simulink library "host_library"  (R2013b)
settings: Solver=ode45  StartTime=0.0  StopTime=10.0  RelTol=1e-3
libraries: embdlinuxlib x9
settings Model: Creator=scastro  LastModifiedBy=scastro

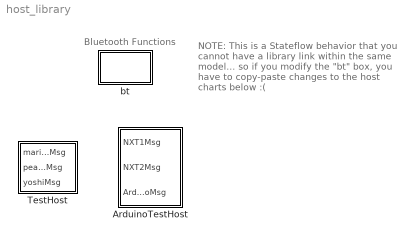
== system host_library ==
  note: NOTE:  This is a Stateflow behavior
      | that you cannot have a library link within the
      | same model... so if you modify the "bt" box,
      | you have to copy-paste changes to the host
      | charts below :(
  note: Bluetooth Functions
  ArduinoTestHost : Stateflow chart  TreatAsAtomicUnit=on
  TestHost : Stateflow chart  TreatAsAtomicUnit=on
  bt : Stateflow chart  TreatAsAtomicUnit=on

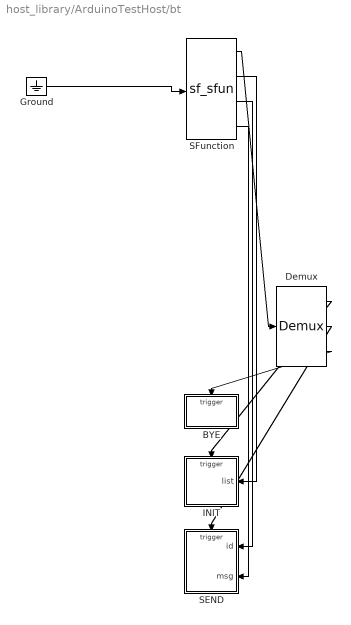
== system host_library/ArduinoTestHost/bt ==
  " Demux " : Demux  Outputs=3
  " Ground " : Ground
  " SFunction " : S-Function  Tag=Stateflow S-Function host_library 4  FunctionName=sf_sfun  PortCounts=[1 4]  EnableBusSupport=off
  BYE : Subsystem
      settings: UndoDeleteFcn=Stateflow.SLINSF.SimulinkMan.restorePreDeleteFcn  PreDeleteFcn=Stateflow.SLINSF.SimulinkMan.removePreDeleteFcn
  INIT : Subsystem
      settings: UndoDeleteFcn=Stateflow.SLINSF.SimulinkMan.restorePreDeleteFcn  PreDeleteFcn=Stateflow.SLINSF.SimulinkMan.removePreDeleteFcn
  SEND : Subsystem
      settings: UndoDeleteFcn=Stateflow.SLINSF.SimulinkMan.restorePreDeleteFcn  PreDeleteFcn=Stateflow.SLINSF.SimulinkMan.removePreDeleteFcn
  wires:
  " SFunction "/1 -> " Demux "/1
  " Ground "/1 -> " SFunction "/1
  " Demux "/3 -> BYE/Trigger
  " Demux "/2 -> SEND/Trigger
  " SFunction "/4 -> SEND/2(msg)
  " SFunction "/3 -> SEND/1(id)
  " Demux "/1 -> INIT/Trigger
  " SFunction "/2 -> INIT/1(list)

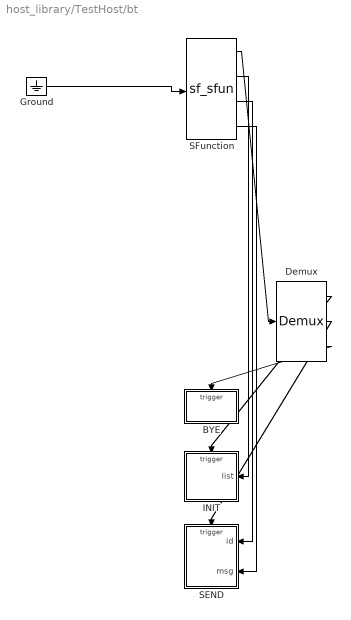
== system host_library/TestHost/bt ==
  " Demux " : Demux  Outputs=3
  " Ground " : Ground
  " SFunction " : S-Function  Tag=Stateflow S-Function host_library 8  FunctionName=sf_sfun  PortCounts=[1 4]  EnableBusSupport=off
  BYE : Subsystem
      settings: UndoDeleteFcn=Stateflow.SLINSF.SimulinkMan.restorePreDeleteFcn  PreDeleteFcn=Stateflow.SLINSF.SimulinkMan.removePreDeleteFcn
  INIT : Subsystem
      settings: UndoDeleteFcn=Stateflow.SLINSF.SimulinkMan.restorePreDeleteFcn  PreDeleteFcn=Stateflow.SLINSF.SimulinkMan.removePreDeleteFcn
  SEND : Subsystem
      settings: UndoDeleteFcn=Stateflow.SLINSF.SimulinkMan.restorePreDeleteFcn  PreDeleteFcn=Stateflow.SLINSF.SimulinkMan.removePreDeleteFcn
  wires:
  " SFunction "/2 -> INIT/1(list)
  " Demux "/1 -> INIT/Trigger
  " SFunction "/3 -> SEND/1(id)
  " SFunction "/4 -> SEND/2(msg)
  " Demux "/2 -> SEND/Trigger
  " Demux "/3 -> BYE/Trigger
  " Ground "/1 -> " SFunction "/1
  " SFunction "/1 -> " Demux "/1

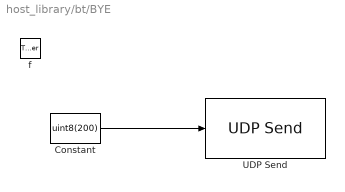
== system host_library/bt/BYE ==
  f : TriggerPort  TriggerType=function-call
      settings: CopyFcn=Stateflow.SLINSF.SimulinkMan.removeBlockPreDeleteFcn  PreDeleteFcn=Stateflow.SLINSF.SimulinkMan.unsafePredeleteFcn
  Constant : Constant  Value=uint8(200)  VectorParams1D=off
      settings: SamplingMode=Frame based
  UDP Send : embdlinuxlib/UDP Send  remoteURL='127.0.0.1'  remotePort=35712  localURL='255.255.255.255'  localPortSource=Automatically determine  localPort=-1  sampletime=-1  blockPlatform=Raspberry Pi  separateLengthPort=0
  wires:
  Constant/1 -> UDP Send/1

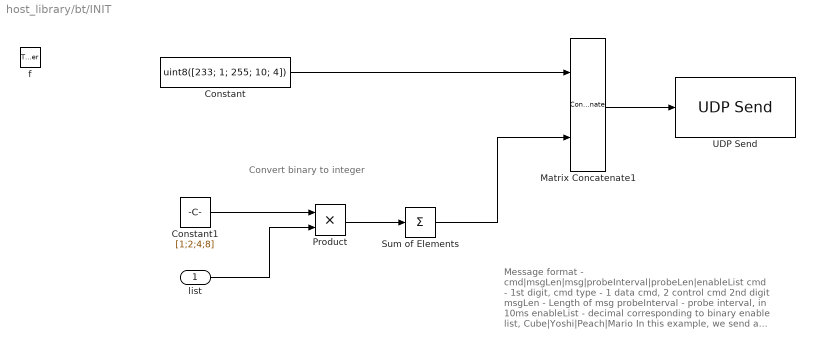
== system host_library/bt/INIT ==
  note: Convert binary to integer
  note: Message format -
      | cmd|msgLen|msg|probeInterval|probeLen|enableList
      | cmd - 1st digit, cmd type - 1 data cmd, 2 control cmd
      | 2nd digit
      | msgLen - Length of msg
      | probeInterval - probe interval, in 10ms
      | enableList - decimal corresponding to binary enable list,
      | Cube|Yoshi|Peach|Mario
      | In this example, we send a unint8 255
  list : Inport  OutDataTypeStr=double  PortDimensions=4
  f : TriggerPort  TriggerType=function-call
      settings: CopyFcn=Stateflow.SLINSF.SimulinkMan.removeBlockPreDeleteFcn  PreDeleteFcn=Stateflow.SLINSF.SimulinkMan.unsafePredeleteFcn
  Constant : Constant  Value=uint8([233; 1; 255; 10; 4])  VectorParams1D=off
      settings: SamplingMode=Frame based
  Constant1 : Constant  Value=[1;2;4;8]
  Matrix Concatenate1 : Concatenate  Mode=Multidimensional array
  Product : Product
  Sum of Elements : Sum  Inputs=+  AccumDataTypeStr=uint8  OutDataTypeStr=uint8
  UDP Send : embdlinuxlib/UDP Send  remoteURL='127.0.0.1'  remotePort=35712  localURL='255.255.255.255'  localPortSource=Automatically determine  localPort=-1  sampletime=-1  blockPlatform=Raspberry Pi  separateLengthPort=0
  wires:
  Matrix Concatenate1/1 -> UDP Send/1
  Constant/1 -> Matrix Concatenate1/1
  Sum of Elements/1 -> Matrix Concatenate1/2
  Product/1 -> Sum of Elements/1
  Constant1/1 -> Product/1
  list/1 -> Product/2

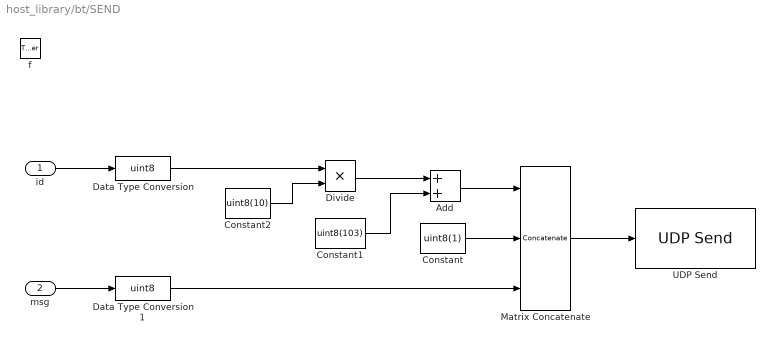
== system host_library/bt/SEND ==
  id : Inport  OutDataTypeStr=Enum: RobotID  PortDimensions=1
  msg : Inport  Port=2  OutDataTypeStr=Enum: StatusID  PortDimensions=1
  f : TriggerPort  TriggerType=function-call
      settings: CopyFcn=Stateflow.SLINSF.SimulinkMan.removeBlockPreDeleteFcn  PreDeleteFcn=Stateflow.SLINSF.SimulinkMan.unsafePredeleteFcn
  Add : Sum
  Constant : Constant  Value=uint8(1)  VectorParams1D=off
  Constant1 : Constant  Value=uint8(103)  VectorParams1D=off
  Constant2 : Constant  Value=uint8(10)  VectorParams1D=off
  Data Type Conversion : DataTypeConversion  OutDataTypeStr=uint8
  Data Type Conversion1 : DataTypeConversion  OutDataTypeStr=uint8
  Divide : Product  Inputs=**  OutDataTypeStr=uint8
  Matrix Concatenate : Concatenate  NumInputs=3  Mode=Multidimensional array
  UDP Send : embdlinuxlib/UDP Send  remoteURL='127.0.0.1'  remotePort=35712  localURL='255.255.255.255'  localPortSource=Automatically determine  localPort=-1  sampletime=-1  blockPlatform=Raspberry Pi  separateLengthPort=0
  wires:
  Matrix Concatenate/1 -> UDP Send/1
  msg/1 -> Data Type Conversion1/1
  Constant/1 -> Matrix Concatenate/2
  Constant2/1 -> Divide/2
  Constant1/1 -> Add/2
  id/1 -> Data Type Conversion/1
  Divide/1 -> Add/1
  Add/1 -> Matrix Concatenate/1
  Data Type Conversion/1 -> Divide/1
  Data Type Conversion1/1 -> Matrix Concatenate/3

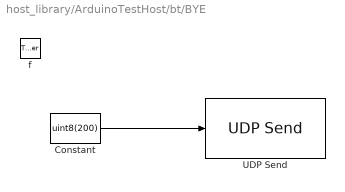
== system host_library/ArduinoTestHost/bt/BYE ==
  f : TriggerPort  TriggerType=function-call
      settings: CopyFcn=Stateflow.SLINSF.SimulinkMan.removeBlockPreDeleteFcn  PreDeleteFcn=Stateflow.SLINSF.SimulinkMan.unsafePredeleteFcn
  Constant : Constant  Value=uint8(200)  VectorParams1D=off
      settings: SamplingMode=Frame based
  UDP Send : embdlinuxlib/UDP Send  remoteURL='127.0.0.1'  remotePort=35712  localURL='255.255.255.255'  localPortSource=Automatically determine  localPort=-1  sampletime=-1  blockPlatform=Raspberry Pi  separateLengthPort=0
  wires:
  Constant/1 -> UDP Send/1

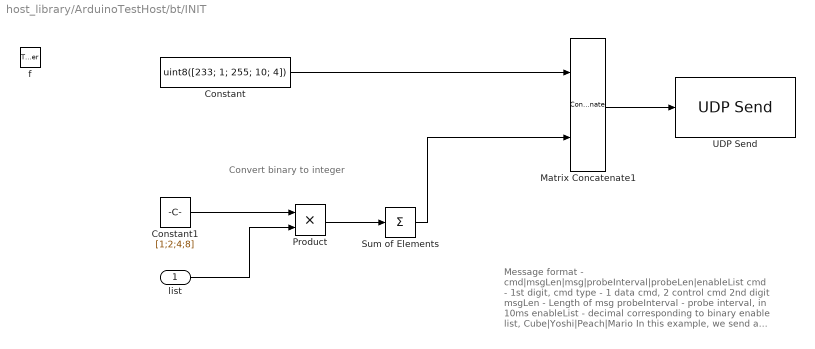
== system host_library/ArduinoTestHost/bt/INIT ==
  note: Convert binary to integer
  note: Message format -
      | cmd|msgLen|msg|probeInterval|probeLen|enableList
      | cmd - 1st digit, cmd type - 1 data cmd, 2 control cmd
      | 2nd digit
      | msgLen - Length of msg
      | probeInterval - probe interval, in 10ms
      | enableList - decimal corresponding to binary enable list,
      | Cube|Yoshi|Peach|Mario
      | In this example, we send a unint8 255
  list : Inport  OutDataTypeStr=double  PortDimensions=4
  f : TriggerPort  TriggerType=function-call
      settings: CopyFcn=Stateflow.SLINSF.SimulinkMan.removeBlockPreDeleteFcn  PreDeleteFcn=Stateflow.SLINSF.SimulinkMan.unsafePredeleteFcn
  Constant : Constant  Value=uint8([233; 1; 255; 10; 4])  VectorParams1D=off
      settings: SamplingMode=Frame based
  Constant1 : Constant  Value=[1;2;4;8]
  Matrix Concatenate1 : Concatenate  Mode=Multidimensional array
  Product : Product
  Sum of Elements : Sum  Inputs=+  AccumDataTypeStr=uint8  OutDataTypeStr=uint8
  UDP Send : embdlinuxlib/UDP Send  remoteURL='127.0.0.1'  remotePort=35712  localURL='255.255.255.255'  localPortSource=Automatically determine  localPort=-1  sampletime=-1  blockPlatform=Raspberry Pi  separateLengthPort=0
  wires:
  list/1 -> Product/2
  Constant1/1 -> Product/1
  Product/1 -> Sum of Elements/1
  Matrix Concatenate1/1 -> UDP Send/1
  Constant/1 -> Matrix Concatenate1/1
  Sum of Elements/1 -> Matrix Concatenate1/2

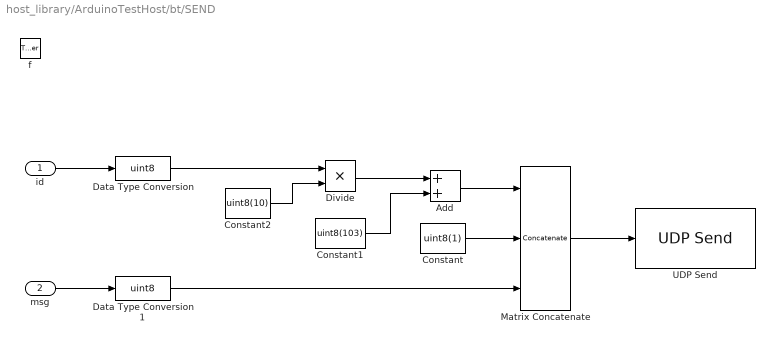
== system host_library/ArduinoTestHost/bt/SEND ==
  id : Inport  OutDataTypeStr=Enum: RobotID  PortDimensions=1
  msg : Inport  Port=2  OutDataTypeStr=Enum: StatusID  PortDimensions=1
  f : TriggerPort  TriggerType=function-call
      settings: CopyFcn=Stateflow.SLINSF.SimulinkMan.removeBlockPreDeleteFcn  PreDeleteFcn=Stateflow.SLINSF.SimulinkMan.unsafePredeleteFcn
  Add : Sum
  Constant : Constant  Value=uint8(1)  VectorParams1D=off
  Constant1 : Constant  Value=uint8(103)  VectorParams1D=off
  Constant2 : Constant  Value=uint8(10)  VectorParams1D=off
  Data Type Conversion : DataTypeConversion  OutDataTypeStr=uint8
  Data Type Conversion1 : DataTypeConversion  OutDataTypeStr=uint8
  Divide : Product  Inputs=**  OutDataTypeStr=uint8
  Matrix Concatenate : Concatenate  NumInputs=3  Mode=Multidimensional array
  UDP Send : embdlinuxlib/UDP Send  remoteURL='127.0.0.1'  remotePort=35712  localURL='255.255.255.255'  localPortSource=Automatically determine  localPort=-1  sampletime=-1  blockPlatform=Raspberry Pi  separateLengthPort=0
  wires:
  Matrix Concatenate/1 -> UDP Send/1
  msg/1 -> Data Type Conversion1/1
  Constant/1 -> Matrix Concatenate/2
  Constant2/1 -> Divide/2
  Constant1/1 -> Add/2
  id/1 -> Data Type Conversion/1
  Divide/1 -> Add/1
  Add/1 -> Matrix Concatenate/1
  Data Type Conversion/1 -> Divide/1
  Data Type Conversion1/1 -> Matrix Concatenate/3

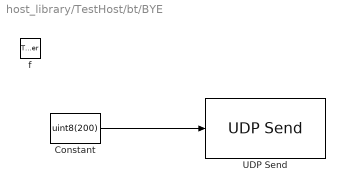
== system host_library/TestHost/bt/BYE ==
  f : TriggerPort  TriggerType=function-call
      settings: CopyFcn=Stateflow.SLINSF.SimulinkMan.removeBlockPreDeleteFcn  PreDeleteFcn=Stateflow.SLINSF.SimulinkMan.unsafePredeleteFcn
  Constant : Constant  Value=uint8(200)  VectorParams1D=off
      settings: SamplingMode=Frame based
  UDP Send : embdlinuxlib/UDP Send  remoteURL='127.0.0.1'  remotePort=35712  localURL='255.255.255.255'  localPortSource=Automatically determine  localPort=-1  sampletime=-1  blockPlatform=Raspberry Pi  separateLengthPort=0
  wires:
  Constant/1 -> UDP Send/1

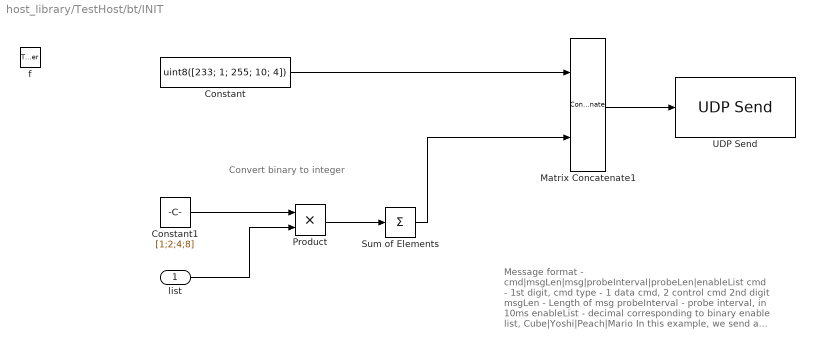
== system host_library/TestHost/bt/INIT ==
  note: Message format -
      | cmd|msgLen|msg|probeInterval|probeLen|enableList
      | cmd - 1st digit, cmd type - 1 data cmd, 2 control cmd
      | 2nd digit
      | msgLen - Length of msg
      | probeInterval - probe interval, in 10ms
      | enableList - decimal corresponding to binary enable list,
      | Cube|Yoshi|Peach|Mario
      | In this example, we send a unint8 255
  note: Convert binary to integer
  list : Inport  OutDataTypeStr=double  PortDimensions=4
  f : TriggerPort  TriggerType=function-call
      settings: CopyFcn=Stateflow.SLINSF.SimulinkMan.removeBlockPreDeleteFcn  PreDeleteFcn=Stateflow.SLINSF.SimulinkMan.unsafePredeleteFcn
  Constant : Constant  Value=uint8([233; 1; 255; 10; 4])  VectorParams1D=off
      settings: SamplingMode=Frame based
  Constant1 : Constant  Value=[1;2;4;8]
  Matrix Concatenate1 : Concatenate  Mode=Multidimensional array
  Product : Product
  Sum of Elements : Sum  Inputs=+  AccumDataTypeStr=uint8  OutDataTypeStr=uint8
  UDP Send : embdlinuxlib/UDP Send  remoteURL='127.0.0.1'  remotePort=35712  localURL='255.255.255.255'  localPortSource=Automatically determine  localPort=-1  sampletime=-1  blockPlatform=Raspberry Pi  separateLengthPort=0
  wires:
  Sum of Elements/1 -> Matrix Concatenate1/2
  Constant/1 -> Matrix Concatenate1/1
  Matrix Concatenate1/1 -> UDP Send/1
  Product/1 -> Sum of Elements/1
  Constant1/1 -> Product/1
  list/1 -> Product/2

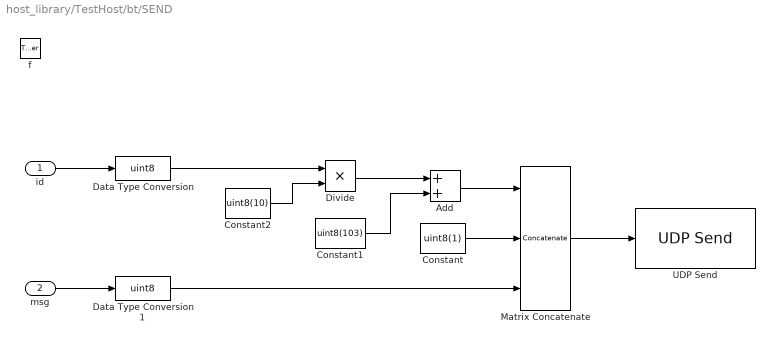
== system host_library/TestHost/bt/SEND ==
  id : Inport  OutDataTypeStr=Enum: RobotID  PortDimensions=1
  msg : Inport  Port=2  OutDataTypeStr=Enum: StatusID  PortDimensions=1
  f : TriggerPort  TriggerType=function-call
      settings: CopyFcn=Stateflow.SLINSF.SimulinkMan.removeBlockPreDeleteFcn  PreDeleteFcn=Stateflow.SLINSF.SimulinkMan.unsafePredeleteFcn
  Add : Sum
  Constant : Constant  Value=uint8(1)  VectorParams1D=off
  Constant1 : Constant  Value=uint8(103)  VectorParams1D=off
  Constant2 : Constant  Value=uint8(10)  VectorParams1D=off
  Data Type Conversion : DataTypeConversion  OutDataTypeStr=uint8
  Data Type Conversion1 : DataTypeConversion  OutDataTypeStr=uint8
  Divide : Product  Inputs=**  OutDataTypeStr=uint8
  Matrix Concatenate : Concatenate  NumInputs=3  Mode=Multidimensional array
  UDP Send : embdlinuxlib/UDP Send  remoteURL='127.0.0.1'  remotePort=35712  localURL='255.255.255.255'  localPortSource=Automatically determine  localPort=-1  sampletime=-1  blockPlatform=Raspberry Pi  separateLengthPort=0
  wires:
  Data Type Conversion1/1 -> Matrix Concatenate/3
  Data Type Conversion/1 -> Divide/1
  Add/1 -> Matrix Concatenate/1
  Divide/1 -> Add/1
  id/1 -> Data Type Conversion/1
  Constant1/1 -> Add/2
  Constant2/1 -> Divide/2
  Constant/1 -> Matrix Concatenate/2
  msg/1 -> Data Type Conversion1/1
  Matrix Concatenate/1 -> UDP Send/1

== stateflow chart host_library/bt ==
  state INIT(list) [function]
  state SEND(id,msg) [function]
  state BYE [function]
  data: list function_input double size=4; id function_input Enum: RobotID size=1; msg function_input Enum: StatusID size=1

== stateflow chart host_library/TestHost ==
  state State1
    en,du:
    bt.SEND(RobotID.MARIO, StatusID.MARIO_ON_SEESAW);
  state bt [group]
  state State2
    en:
    done = true;
  (default) -> State1
  State1 -> State2 : after(10,sec)
  data: marioMsg input; peachMsg input; yoshiMsg input; done data_store_memory

== stateflow chart host_library/ArduinoTestHost ==
  state State1
  state bt [group]
  state State2
    en:
    bt.SEND(RobotID.NXT1, StatusID.NXT1_GO_DOWN_RAMP);
  state State3
    en:
    done = true;
  (default) -> State1
  State1 -> State3 [order 2] : after(240,sec)
  State1 -> State2 [order 1] : [isequal(ArduinoMsg,StatusID.ROVER_SENSED_RAMP)]
  State2 -> State3 : after(10,sec)
  data: NXT1Msg input; NXT2Msg input; ArduinoMsg input; done data_store_memory

== stateflow chart host_library/ArduinoTestHost/bt ==
  state INIT(list) [function]
  state SEND(id,msg) [function]
  state BYE [function]
  data: list function_input double size=4; id function_input Enum: RobotID size=1; msg function_input Enum: StatusID size=1

== stateflow chart host_library/TestHost/bt ==
  state INIT(list) [function]
  state SEND(id,msg) [function]
  state BYE [function]
  data: list function_input double size=4; id function_input Enum: RobotID size=1; msg function_input Enum: StatusID size=1
